simulink model "DM"  (R2020a)
settings: Solver=VariableStepAuto  StartTime=0.0  StopTime=20  RelTol=1e-3
settings Model: Creator=Admin  LastModifiedBy=fazal
settings SFSimCC: CustomCodeUndefinedFunction=UseInterfaceOnly

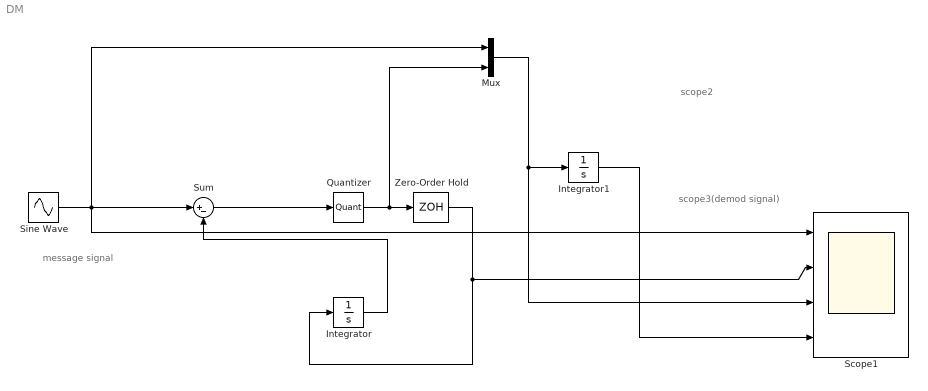
== system DM ==
  note: scope3(demod signal)
  note: scope2
  note: message signal
  Integrator : Integrator
  Integrator1 : Integrator
  Mux : Mux  Inputs=2
  Quantizer : Quantizer
  Scope1 : Scope  NumInputPorts=4
  Sine Wave : Sin  SampleTime=0
  Sum : Sum  Inputs=|+-
  Zero-Order Hold : ZeroOrderHold  SampleTime=-1
  wires:
  Sine Wave/1 -> Scope1/1, Mux/1, Sum/1
  Sum/1 -> Quantizer/1
  Quantizer/1 -> Mux/2, Zero-Order Hold/1
  Integrator/1 -> Sum/2
  Zero-Order Hold/1 -> Integrator/1, Scope1/2
  Mux/1 -> Scope1/3, Integrator1/1
  Integrator1/1 -> Scope1/4
